simulink model "OEdiff2RTN"  (R2023a)
settings: Solver=ode4  StartTime=0.0  StopTime=10.0  FixedStep=dt  RelTol=1e-3
settings Model: Creator=ndelurgio  LastModifiedBy=ndelurgio

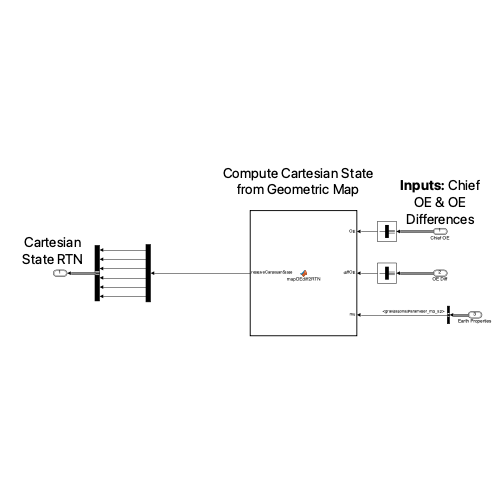
[thumbnail: Simulink's stored preview of the top-level diagram]
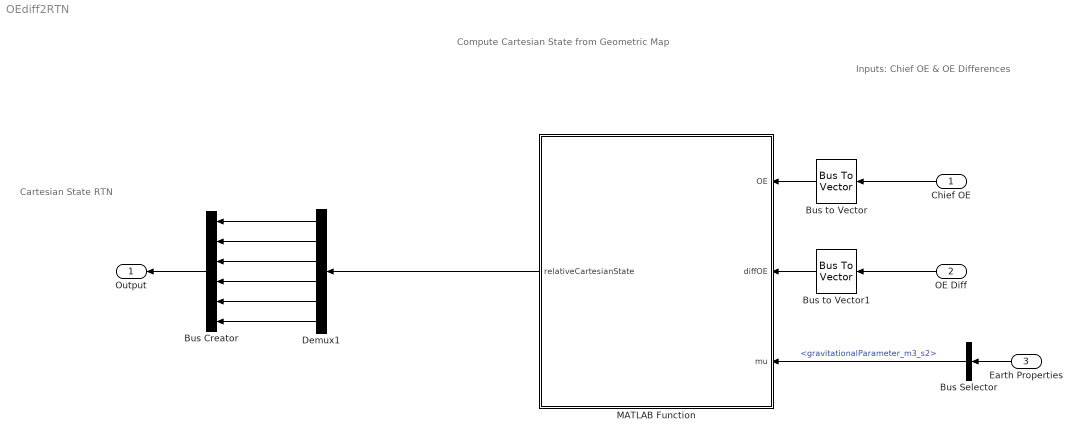
== system OEdiff2RTN ==
  note: Compute Cartesian State from Geometric Map
  note: Inputs: Chief OE & OE Differences
  note: Cartesian State RTN
  Chief OE : Inport  OutDataTypeStr=Bus: osculatingOrbitElements
  OE Diff : Inport  Port=2  OutDataTypeStr=Bus: orbitElementDifferences
  Earth Properties : Inport  Port=3  OutDataTypeStr=Bus: earthProperties
  Bus Creator : BusCreator  Inputs=6  OutDataTypeStr=Bus: relativeCartesianState
      settings: InheritFromInputs=off
  Bus Selector : BusSelector  OutputSignals=gravitationalParameter_m3_s2
  Bus to Vector : BusToVector
  Bus to Vector1 : BusToVector
  Demux1 : Demux  Outputs=6
  MATLAB Function : MATLAB Function  TreatAsAtomicUnit=on
  Output : Outport  OutDataTypeStr=Bus: relativeCartesianState
  wires:
  Chief OE/1 -> Bus to Vector/1
  OE Diff/1 -> Bus to Vector1/1
  Bus to Vector/1 -> MATLAB Function/1(OE)
  Bus to Vector1/1 -> MATLAB Function/2(diffOE)
  MATLAB Function/1(relativeCartesianState) -> Demux1/1
  Demux1/1 -> Bus Creator/1
  Demux1/2 -> Bus Creator/2
  Demux1/3 -> Bus Creator/3
  Demux1/4 -> Bus Creator/4
  Demux1/5 -> Bus Creator/5
  Demux1/6 -> Bus Creator/6
  Bus Creator/1 -> Output/1
  Earth Properties/1 -> Bus Selector/1
  Bus Selector/1 -> MATLAB Function/3(mu)  "<gravitationalParameter_m3_s2>"

== matlab function OEdiff2RTN/MATLAB Function ==
  data: OE input; diffOE input; relativeCartesianState output; mu input
function relativeCartesianState = mapOEdiff2RTN(OE,diffOE,mu)
relativeCartesianState = mapOEdiff2RTN(diffOE,OE,mu);
end
